simulink model "enabled_and_triggered"  (R2024a)
settings: Solver=VariableStepAuto  StartTime=0.0  StopTime=6  RelTol=1e-3  EnableMultiTasking=on
settings Model: Creator=nicholas  LastModifiedBy=bneiswan
settings SolverCC: AlgebraicLoopSolver=TrustRegion
settings DataIOCC: LimitDataPoints=on  SignalLoggingName=logsOut
settings OptimizationCC: BooleanDataType=off  ReuseModelBlockBuffer=off  ExpressionDepthLimit=2147483647  InitFltsAndDblsToZero=on  LifeSpan=inf
settings DebuggingCC: UnconnectedInputMsg=warning  UnconnectedOutputMsg=warning  UnconnectedLineMsg=warning  PregeneratedLibrarySubsystemCodeDiagnostic=none  SubsystemReferenceDiagnosticForUnitTest=warning
settings HardwareCC: ProdBitPerPointer=32  ProdBitPerSizeT=32  ProdBitPerPtrDiffT=32  ProdLargestAtomicFloat=None  ProdIntDivRoundTo=Undefined  ProdEndianess=Unspecified  ProdWordSize=32  ProdHWDeviceType=32-bit Generic  TargetUnknown=on
settings ModelReferenceCC: EnableRefExpFcnMdlSchedulingChecks=on  PropagateSignalLabelsOutOfModel=off
settings SFSimCC: SimUseLocalCustomCode=off
settings RTWCC: RTWUseLocalCustomCode=off  GPUComputeCapability=3.5  DLArmComputeVersion=19.05
settings CodeAppCC: StateflowObjectComments=on
settings GRTTargetCC: TargetFcnLib=ansi_tfl_tmw.mat  TargetLangStandard=C89/C90 (ANSI)  CombineOutputUpdateFcns=off  GRTInterface=on
settings ConfigComp: CovMetricSettings=dw  CovSaveCumulativeToWorkspaceVar=on  CovSaveSingleToWorkspaceVar=on  CovExternalEMLEnable=off  CovSFcnEnable=off

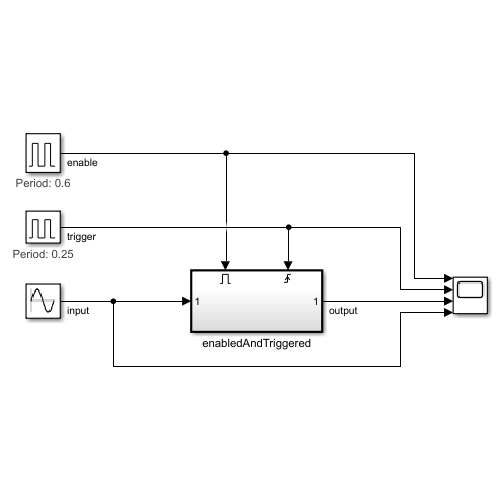
[thumbnail: Simulink's stored preview of the top-level diagram]
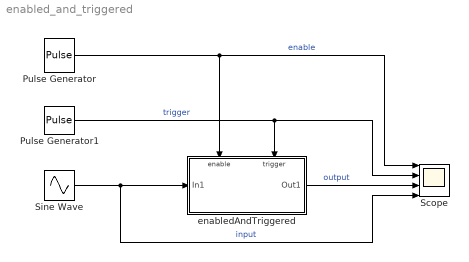
== system enabled_and_triggered ==
  Pulse Generator : DiscretePulseGenerator  PulseType=Time based  Period=0.6  PulseWidth=50
      settings: AttributesFormatString=Period: %<Period>
  Pulse Generator1 : DiscretePulseGenerator  PulseType=Time based  Period=0.25  PulseWidth=50
      settings: AttributesFormatString=Period: %<Period>
  Scope : Scope  NumInputPorts=4
  Sine Wave : Sin  SampleTime=0
  enabledAndTriggered : Subsystem  TreatAsAtomicUnit=on
  wires:
  Sine Wave/1 -> enabledAndTriggered/1(In1), Scope/4  "input"
  Pulse Generator/1 -> Scope/1, enabledAndTriggered/Enable  "enable"
  enabledAndTriggered/1(Out1) -> Scope/3  "output"
  Pulse Generator1/1 -> Scope/2, enabledAndTriggered/Trigger  "trigger"

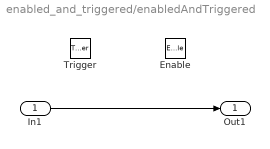
== system enabled_and_triggered/enabledAndTriggered ==
  In1 : Inport
  Enable : EnablePort  StatesWhenEnabling=reset
  Trigger : TriggerPort  VariantControl=Variant
  Out1 : Outport  OutputWhenDisabled=reset  InitialOutput=[0]  VectorParamsAs1DForOutWhenUnconnected=off
  wires:
  In1/1 -> Out1/1
